simulink model "deng_feng_unpack"  (R2016b)
(part 3 of 28)

  pipeline10/1(q) -> Gateway Out1/1, [unpack_sync]
  pipeline11/1(q) -> Gateway Out2/1, [unpack_d160]
  pipeline12/1(q) -> Gateway Out3/1, [unpack_dv]
  pipeline15/1(q) -> Gateway Out4/1, [unpack_timestamp]
  Constant1/1 -> sync_gen/4(misci)
  pipeline59/1(q) -> [ct_tvg_en]
  control/11(in_ct_tvg_en) -> pipeline59/1(d)
  pipeline52/1(q) -> [up_dbg_rst]
  control/12(in_unpack_debug_reset) -> pipeline52/1(d)
  control/13(in_cd_bypass) -> pipeline131/1(d)
  pipeline131/1(q) -> [cd_bypass]
  Concat22/1 -> [ld_val0]
  Concat3/1 -> [ld_val1]
  phase0/1(in_initial) -> Reinterpret2/1
  delta_delay0/1(in_delta) -> Reinterpret1/1
  phase0/2(in_delta) -> Reinterpret3/1
  Reinterpret8/1 -> Concat22/1
  Reinterpret1/1 -> Concat22/2
  Reinterpret2/1 -> Concat22/3
  Reinterpret3/1 -> Concat22/4
  phase1/1(in_initial) -> Reinterpret5/1
  delta_delay1/1(in_delta) -> Reinterpret4/1
  phase1/2(in_delta) -> Reinterpret6/1
  Reinterpret4/1 -> Concat3/2
  Reinterpret5/1 -> Concat3/3
  Reinterpret6/1 -> Concat3/4
  Reinterpret7/1 -> Concat3/1
  delay0/1(in_initial) -> Reinterpret8/1
  delay1/1(in_initial) -> Reinterpret7/1
  pipeline93/1(q) -> [tvg_adc1_en]
  control/6(in_tvg_adc1) -> pipeline93/1(d)
  control/14(in_gbe_stopmux) -> pipeline9/1(d)
  pipeline9/1(q) -> [gbe_stopmux]
  control/15(in_pfb_bypass) -> pipeline66/1(d)
  pipeline66/1(q) -> [pfb_bypass]
  ts_tvg/1(sync) -> pipeline10/1(d)
  ts_tvg/2(d160) -> pipeline11/1(d)
  ts_tvg/3(dv) -> pipeline12/1(d)
  ts_tvg/4(time) -> pipeline15/1(d)
  ts_tvg/5(recvd) -> Terminator9/1
  control/16(in_ts_tvg_en) -> pipeline148/1(d)
  pipeline148/1(q) -> [ts_tvg_en]
  [ts_tvg_en] -> Gateway Out5/1, ts_tvg/1(tvg_en)
  Constant55/1 -> control/5(sim_5)
  Constant56/1 -> control/6(sim_6)
  Constant57/1 -> control/7(sim_7)
  Constant58/1 -> control/8(sim_8)
  Constant59/1 -> control/11(sim_11)
  Constant60/1 -> control/12(sim_12)
  Constant61/1 -> control/13(sim_13)
  Constant62/1 -> control/16(sim_16)
  Constant63/1 -> control/4(sim_4)
  Constant64/1 -> control/3(sim_3)
  Constant65/1 -> control/2(sim_2)
  Constant66/1 -> control/1(sim_1)
  Constant67/1 -> control/9(sim_9)
  Constant68/1 -> control/10(sim_10)
  Constant69/1 -> control/15(sim_15)
  Constant70/1 -> control/14(sim_14)
  impulse_gen0/1(sync_out) -> Gateway Out7/1, [sync80]
  Constant72/1 -> impulse0/1(sim_1)
  Constant73/1 -> impulse0/2(sim_2)
  [unpack_timestamp] -> Concat9/1
  Gateway Out1/1 -> To Workspace1/1
  Gateway Out2/1 -> To Workspace2/1
  Gateway Out3/1 -> To Workspace3/1
  Gateway Out4/1 -> To Workspace4/1
  Gateway Out5/1 -> To Workspace5/1
  Gateway Out6/1 -> To Workspace6/1
  Gateway Out8/1 -> To Workspace8/1
  Gateway Out9/1 -> To Workspace9/1
  Gateway Out10/1 -> To Workspace10/1
  Gateway Out11/1 -> To Workspace11/1
  [up_timestep_error] -> Terminator2/1
  [sys_rst] -> Logical15/1, Logical15/2
  Gateway Out38/1 -> To Workspace30/1
  [sys_relock] -> Gateway Out38/1
  Gateway Out7/1 -> To Workspace7/1
  Gateway Out12/1 -> To Workspace12/1
  Gateway Out86/1 -> To Workspace85/1
  Gateway Out87/1 -> To Workspace86/1
  Constant4/1 -> [Start_Stop_Sel]
  Constant6/1 -> [Impulse_gen0]
  Gateway Out88/1 -> To Workspace88/1
  Gateway Out89/1 -> To Workspace89/1
  Gateway Out13/1 -> To Workspace13/1
  Gateway Out14/1 -> To Workspace14/1
  Gateway Out15/1 -> To Workspace15/1
  Gateway Out16/1 -> To Workspace16/1
  Gateway Out17/1 -> To Workspace17/1
  Delay109/1 -> Gateway Out17/1, Mux12/1
  Gateway Out18/1 -> To Workspace18/1
  Gateway Out19/1 -> To Workspace19/1
  Gateway Out20/1 -> To Workspace20/1
  munge/1(dout) -> [sp256_data], Gateway Out54/1
  Gateway Out21/1 -> To Workspace21/1
  bus_expand/1(msb_out8) -> Gateway Out21/1
  Gateway Out22/1 -> To Workspace22/1
  bus_expand/2(out7) -> Gateway Out22/1
  Gateway Out23/1 -> To Workspace23/1
  bus_expand/3(out6) -> Gateway Out23/1
  Gateway Out24/1 -> To Workspace24/1
  bus_expand/4(out5) -> Gateway Out24/1
  Gateway Out25/1 -> To Workspace25/1
  bus_expand/5(out4) -> Gateway Out25/1
  Gateway Out26/1 -> To Workspace26/1
  bus_expand/6(out3) -> Gateway Out26/1
  Gateway Out27/1 -> To Workspace27/1
  bus_expand/7(out2) -> Gateway Out27/1
  Gateway Out28/1 -> To Workspace28/1
  bus_expand/8(lsb_out1) -> Gateway Out28/1
  Gateway Out29/1 -> To Workspace29/1
  Gateway Out30/1 -> To Workspace31/1
  Gateway Out31/1 -> To Workspace32/1
  bus_expand1/1(msb_out8) -> Gateway Out31/1
  Gateway Out32/1 -> To Workspace33/1
  bus_expand1/2(out7) -> Gateway Out32/1
  Gateway Out33/1 -> To Workspace34/1
  bus_expand1/3(out6) -> Gateway Out33/1
  Gateway Out34/1 -> To Workspace35/1
  bus_expand1/4(out5) -> Gateway Out34/1
  Gateway Out35/1 -> To Workspace36/1
  bus_expand1/5(out4) -> Gateway Out35/1
  Gateway Out37/1 -> To Workspace37/1
  bus_expand1/6(out3) -> Gateway Out37/1
  Gateway Out39/1 -> To Workspace38/1
  bus_expand1/7(out2) -> Gateway Out39/1
  Gateway Out40/1 -> To Workspace39/1
  bus_expand1/8(lsb_out1) -> Gateway Out40/1
  [data_80_tp] -> bus_expand1/1(bus_in)
  Gateway Out41/1 -> To Workspace40/1
  pipeline446/1(q) -> [rdy0], spead_pack4/1(data64_ready)  "rdy0"
  Gateway Out42/1 -> To Workspace41/1
  Gateway Out43/1 -> To Workspace42/1
  Gateway Out44/1 -> To Workspace43/1
  [sp256_data] -> unpack_and_reorder/1(d256)
  [sp256_dv] -> unpack_and_reorder/2(dv256)
  [sp256_eof] -> unpack_and_reorder/3(eof256)
  Gateway Out45/1 -> To Workspace44/1
  Gateway Out46/1 -> To Workspace45/1
  Gateway Out47/1 -> To Workspace46/1
  Gateway Out48/1 -> To Workspace47/1
  Gateway Out49/1 -> To Workspace48/1
  Gateway Out50/1 -> To Workspace49/1
  Gateway Out51/1 -> To Workspace50/1
  Gateway Out52/1 -> To Workspace51/1
  Gateway Out53/1 -> To Workspace52/1
  Gateway Out54/1 -> To Workspace53/1
  Gateway Out55/1 -> To Workspace59/1
  Gateway Out56/1 -> To Workspace60/1
  Gateway Out57/1 -> To Workspace61/1
  Gateway Out58/1 -> To Workspace57/1
  [sp256_dv2] -> Terminator7/1  "dv2"
  [rdy0] -> Gateway Out41/1
  [vld0] -> Gateway Out42/1
  Gateway Out59/1 -> To Workspace54/1
  Gateway Out60/1 -> To Workspace55/1
  [rdy1] -> Gateway Out59/1
  [vld1] -> Gateway Out60/1
  Gateway Out61/1 -> To Workspace56/1
  Gateway Out62/1 -> To Workspace58/1
  [rdy2] -> Gateway Out61/1
  [vld2] -> Gateway Out62/1
  Gateway Out63/1 -> To Workspace62/1
  Gateway Out64/1 -> To Workspace63/1
  [rdy3] -> Gateway Out63/1
  [vld3] -> Gateway Out64/1
  pipeline270/1(q) -> [sp256_data0]
  pipeline371/1(q) -> [sp256_data1]
  pipeline365/1(q) -> [sp256_data2]
  pipeline378/1(q) -> [sp256_data3]
  Gateway Out65/1 -> To Workspace64/1
  bus_expand3/1(msb_out8) -> Gateway Out65/1
  Gateway Out66/1 -> To Workspace65/1
  bus_expand3/2(out7) -> Gateway Out66/1
  Gateway Out67/1 -> To Workspace66/1
  bus_expand3/3(out6) -> Gateway Out67/1
  Gateway Out68/1 -> To Workspace67/1
  bus_expand3/4(out5) -> Gateway Out68/1
  Gateway Out69/1 -> To Workspace68/1
  bus_expand3/5(out4) -> Gateway Out69/1
  Gateway Out70/1 -> To Workspace69/1
  bus_expand3/6(out3) -> Gateway Out70/1
  Gateway Out71/1 -> To Workspace70/1
  bus_expand3/7(out2) -> Gateway Out71/1
  Gateway Out72/1 -> To Workspace71/1
  bus_expand3/8(lsb_out1) -> Gateway Out72/1
  bus_expand2/1(msb_out2) -> bus_expand3/1(bus_in)
  Gateway Out73/1 -> To Workspace72/1
  bus_expand4/1(msb_out8) -> Gateway Out73/1
  Gateway Out74/1 -> To Workspace73/1
  bus_expand4/2(out7) -> Gateway Out74/1
  Gateway Out75/1 -> To Workspace74/1
  bus_expand4/3(out6) -> Gateway Out75/1
  Gateway Out76/1 -> To Workspace75/1
  bus_expand4/4(out5) -> Gateway Out76/1
  Gateway Out77/1 -> To Workspace76/1
  bus_expand4/5(out4) -> Gateway Out77/1
  Gateway Out78/1 -> To Workspace77/1
  bus_expand4/6(out3) -> Gateway Out78/1
  Gateway Out79/1 -> To Workspace78/1
  bus_expand4/7(out2) -> Gateway Out79/1
  Gateway Out80/1 -> To Workspace79/1
  bus_expand4/8(lsb_out1) -> Gateway Out80/1
  bus_expand2/2(lsb_out1) -> bus_expand4/1(bus_in)
  Gateway Out81/1 -> To Workspace80/1
  bus_expand7/1(msb_out8) -> Gateway Out81/1
  Gateway Out82/1 -> To Workspace81/1
  bus_expand7/2(out7) -> Gateway Out82/1
  Gateway Out83/1 -> To Workspace82/1
  bus_expand7/3(out6) -> Gateway Out83/1
  Gateway Out84/1 -> To Workspace83/1
  bus_expand7/4(out5) -> Gateway Out84/1
  Gateway Out85/1 -> To Workspace84/1
  bus_expand7/5(out4) -> Gateway Out85/1
  Gateway Out90/1 -> To Workspace87/1
  bus_expand7/6(out3) -> Gateway Out90/1
  Gateway Out91/1 -> To Workspace90/1
  bus_expand7/7(out2) -> Gateway Out91/1
  Gateway Out92/1 -> To Workspace91/1
  bus_expand7/8(lsb_out1) -> Gateway Out92/1
  bus_expand5/1(msb_out2) -> bus_expand7/1(bus_in)
  Gateway Out93/1 -> To Workspace92/1
  bus_expand8/1(msb_out8) -> Gateway Out93/1
  Gateway Out94/1 -> To Workspace93/1
  bus_expand8/2(out7) -> Gateway Out94/1
  Gateway Out95/1 -> To Workspace94/1
  bus_expand8/3(out6) -> Gateway Out95/1
  Gateway Out96/1 -> To Workspace95/1
  bus_expand8/4(out5) -> Gateway Out96/1
  Gateway Out97/1 -> To Workspace96/1
  bus_expand8/5(out4) -> Gateway Out97/1
  Gateway Out98/1 -> To Workspace97/1
  bus_expand8/6(out3) -> Gateway Out98/1
  Gateway Out99/1 -> To Workspace98/1
  bus_expand8/7(out2) -> Gateway Out99/1
  Gateway Out100/1 -> To Workspace99/1
  bus_expand8/8(lsb_out1) -> Gateway Out100/1
  bus_expand5/2(lsb_out1) -> bus_expand8/1(bus_in)
  unpack_and_reorder/2(d160) -> bus_expand5/1(bus_in), Gateway Out8/1, ts_tvg/3(data_in)
